simulink model "robot_continuous"  (R2024a)
settings: Solver=FixedStepAuto  StartTime=0.0  StopTime=50  FixedStep=0.0005  RelTol=1e-3
settings Model: Creator=YAO_H  LastModifiedBy=YAO_H
settings DataIOCC: SaveFinalState=on  SaveOperatingPoint=on

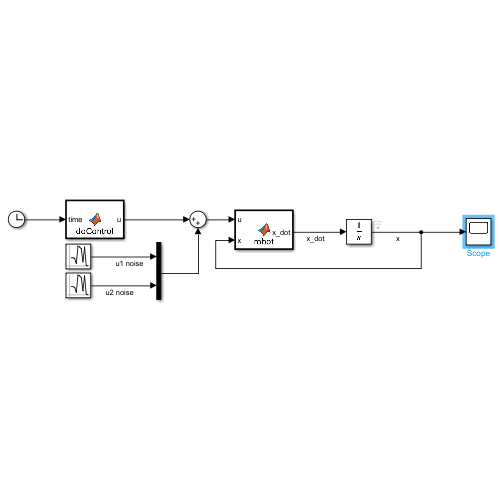
[thumbnail: Simulink's stored preview of the top-level diagram]
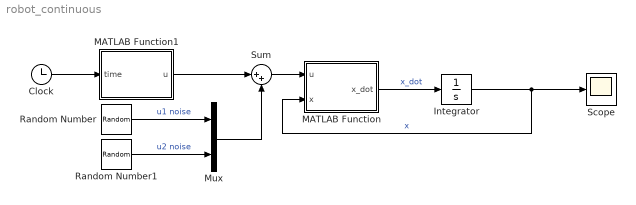
== system robot_continuous ==
  Clock : Clock
  Integrator : Integrator  InitialCondition=[0;0;0]
  MATLAB Function : MATLAB Function  TreatAsAtomicUnit=on
  MATLAB Function1 : MATLAB Function  TreatAsAtomicUnit=on
  Mux : Mux  Inputs=2
  Random Number : RandomNumber  SampleTime=0.0005
  Random Number1 : RandomNumber  Variance=0.01  SampleTime=0.0005
  Scope : Scope
  Sum : Sum  Inputs=|++
  wires:
  Integrator/1 -> Scope/1, MATLAB Function/2(x)  "x"
  MATLAB Function/1(x_dot) -> Integrator/1  "x_dot"
  Clock/1 -> MATLAB Function1/1(time)
  Sum/1 -> MATLAB Function/1(u)
  Mux/1 -> Sum/2
  Random Number/1 -> Mux/1  "u1 noise"
  MATLAB Function1/1(u) -> Sum/1
  Random Number1/1 -> Mux/2  "u2 noise"

== matlab function robot_continuous/MATLAB Function ==
  data: u input; x_dot output; x input
function x_dot = robot(u, x)
    s = u(1);  % 线速度 (m/s)
    omega = u(2);  % 角速度 (rad/s)
    theta = x(3);  % 取当前角度
    
    % 计算微分方程
    x_dot = [s * cos(theta);
             s * sin(theta);
             omega];
end

== matlab function robot_continuous/MATLAB Function1 ==
  data: time input; u output
function u = doControl(time)
    T = 10;  % time constant
    V = 0.1; 
    yawrate = 5 * pi / 180;
    u = [ V * (1 - exp(-time/T)); yawrate * (1 - exp(-time/T)) ];
end
